simulink model "wlan_mac_hw"  (Simulink 7.8)
settings: Solver=ode45  StartTime=0.0  StopTime=200  RelTol=1e-3
PostLoadFcn:
  | wlan_mac_hw_init
InitFcn:
  | wlan_mac_hw_init
StartFcn:
  | wlan_mac_hw_init
values from neighbouring files (symbols this model uses):
  NB_CNTR_NAV = ceil(log2(MAX_NAV * 160))    [wlan_mac_hw_init.m]
  ticks_per_usec = 10    [wlan_mac_hw_init.m]
undefined symbols (not defined in the file or in its folder): gcbh, xlBlockLoadCallback, xlGetNormalizedPeriod
libraries: xbsIndex_r4 x788, xbsEDKLib_r4 x1
(part 1 of 6)
settings Model: Creator=murphpo  LastModifiedBy=murphpo
settings DebuggingCC: SolverPrmCheckMsg=none  InheritedTsInSrcMsg=none  UnconnectedInputMsg=none  UnconnectedOutputMsg=none  UnconnectedLineMsg=none

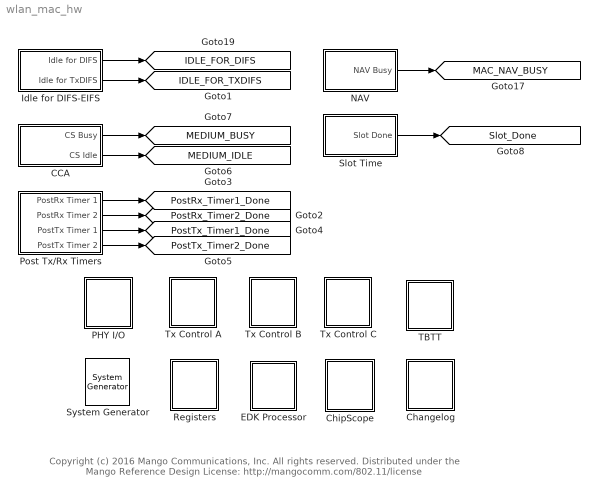
== system wlan_mac_hw ==
  note: Copyright (c) 2016 Mango Communications, Inc. All rights reserved.
      |
      | Distributed under the Mango Reference Design License:
      | http://mangocomm.com/802.11/license
  " System Generator" : xbsIndex_r4/ System Generator  Tag=genX  xilinxfamily=virtex6  part=xc6vlx240t  speed=-2  package=ff1156  synthesis_tool=XST  clock_wrapper=Clock Enables  directory=./pcore_v212  proj_type=Project Navigator  Synth_file=XST Defaults  Impl_file=ISE Defaults  testbench=off  simulink_period=1  sysclk_period=10  dcm_input_clock_period=10  incr_netlist=off  trim_vbits=Everywhere in SubSystem  dbl_ovrd=According to Block Masks  core_generation=According to Block Masks  run_coregen=off  deprecated_control=off  eval_field=0  block_type=sysgen
  CCA : Subsystem
  Changelog : Subsystem
  ChipScope : Subsystem
  EDK Processor : Subsystem  LoadFcn=xlBlockLoadCallback(gcbh);  mask(Xilinx EDK Processor Block){mode=EDK pcore generation, xmp=, MemVisToProc=<qt bgcolor="#FFFFFF"><div><img src="S:/Xilinx/14.4/ISE_DS/ISE/sysgen/data/images/registerplus.gif"> &lt;&lt;TX_CTRL_B_PARAMS&gt;&gt;<br></div><div><img src="S:/Xilinx/14.4/ISE_DS/ISE/sysgen/data/images/registerplus.gif"> &lt;&lt;TX_CTRL_A_GAINS&gt;&gt;<br></div><div><img src="S:/Xilinx/14.4/ISE_DS/ISE/sysgen/data/images/registerplus.gif"> &lt;&lt;TX_CTRL_C_PARAMS&gt;&gt;<br></div><div><img src="S:/Xilinx/14.4/ISE_DS/ISE/sysgen/data/images/registerplus.gif"> &lt;&lt;TX_CTRL_A_PARAMS&gt;&gt;<br></div><div><img src="S:/Xilinx/14.4/ISE_DS/ISE/sysgen/data/images/registerplus.gif"> &lt;&lt;TX_CTRL_C_GAINS&gt;&gt;<br></div><div><img src="S:/Xilinx/14.4/ISE_DS/ISE/sysgen/data/images/registerplus.gif"> &lt;&lt;POST_RX_TIMERS&gt;&gt;<br></div><div><img src="S:/Xilinx/14.4/ISE_DS/ISE/sysgen/data/images/registerplus.gif"> &lt;&lt;TX_CTRL_B_GAINS&gt;&gt;<br></div><div><img src="S:/Xilinx/14.4/ISE_DS/ISE/sysgen/data/images/registerplus.gif"> &lt;&lt;POST_TX_TIMERS&gt;&gt;<br></div><div><img src="S:/Xilinx/14.4/ISE_DS/ISE/sysgen/data/images/registerplus.gif"> &lt;&lt;CALIB_TIMES&gt;&gt;<br></div><div><img src="S:/Xilinx/14.4/ISE_DS/ISE/sysgen/data/images/registerplus.gif"> &lt;&lt;IFS_INTERVALS2&gt;&gt;<br></div><div><img src="S:/Xilinx/14.4/ISE_DS/ISE/sysgen/data/images/registerplus.gif"> &lt;&lt;IFS_INTERVALS1&gt;&gt;<br></div><div><img src="S:/Xilinx/14.4/ISE_DS/ISE/sysgen/data/images/registerplus.gif"> &lt;&lt;TX_START&gt;&gt;<br></div><div><img src="S:/Xilinx/14.4/ISE_DS/ISE/sysgen/data/images/registerplus.gif"> &lt;&lt;TU_TARGET&gt;&gt;<br></div><div><img src="S:/Xilinx/14.4/ISE_DS/ISE/sysgen/data/images/registerplus.gif"> &lt;&lt;Control&gt;&gt;<br></div><div><img src="S:/Xilinx/14.4/ISE_DS/ISE/sysgen/data/images/registerplus.gif"> &lt;&lt;NAV_MATCH_ADDR_1&gt;&gt;<br></div><div><img src="S:/Xilinx/14.4/ISE_DS/ISE/sysgen/data/images/registerplus.gif"> &lt;&lt;NAV_MATCH_ADDR_2&gt;&gt;<br></div><div><img src="S:/Xilinx/14.4/ISE_DS/ISE/sysgen/data/images/registerplus.gif"> &lt;&lt;BACKOFF_CTRL&gt;&gt;<br></div><div><img src="S:/Xilinx/14.4/ISE_DS/ISE/sysgen/data/images/registerplus.gif"> &lt;&lt;NAV_VALUE&gt;&gt;<br></div><div><img src="S:/Xilinx/14.4/ISE_DS/ISE/sysgen/data/images/registerplus.gif"> &lt;&lt;BACKOFF_COUNTERS&gt;&gt;<br></div><div><img src="S:/Xilinx/14.4/ISE_DS/ISE/sysgen/data/images/registerplus.gif"> &lt;&lt;PHY_RX_PARAMS&gt;&gt;<br></div><div><img src="S:/Xilinx/14.4/ISE_DS/ISE/sysgen/data/images/registerplus.gif"> &lt;&lt;LATEST_RX_BYTE&gt;&gt;<br></div><div><img src="S:/Xilinx/14.4/ISE_DS/ISE/sysgen/data/images/registerplus.gif"> &lt;&lt;TX_START_TIMESTAMP_MSB&gt;&gt;<br></div><div><img src="S:/Xilinx/14.4/ISE_DS/ISE/sysgen/data/images/registerplus.gif"> &lt;&lt;TX_START_TIMESTAMP_LSB&gt;&gt;<br></div><div><img src="S:/Xilinx/14.4/ISE_DS/ISE/sysgen/data/images/registerplus.gif"> &lt;&lt;RX_START_TIMESTAMP_MSB&gt;&gt;<br></div><div><img src="S:/Xilinx/14.4/ISE_DS/ISE/sysgen/data/images/registerplus.gif"> &lt;&lt;RX_START_TIMESTAMP_LSB&gt;&gt;<br></div><div><img src="S:/Xilinx/14.4/ISE_DS/ISE/sysgen/data/images/registerplus.gif"> &lt;&lt;TXRX_START_TIMESTAMPS_FRAC&gt;&gt;<br></div><div><img src="S:/Xilinx/14.4/ISE_DS/ISE/sysgen/data/images/registerplus.gif"> &lt;&lt;Status&gt;&gt;<br></div></qt>, AvailableMemories=<empty>, portInterfaceTable={'exposed'=>[],'portdir'=>[],'portname'=>[],'shortname'=>[]}, bus_type_sgadvanced=, bus_type=AXI, baseaddr=0x80000000, baseaddr_lock_sgadvanced=, baseaddr_lock=off, dual_clock_sgadvanced=, dual_clock=on, reg_readback_sgadvanced=, reg_readback=on, ucf_file=, inheritDeviceType_sgadvanced=, inheritDeviceType=off, elf_file=, codebug_sgadvanced=, codebug=on, clock_name=plb, internalPortList={}, resetPolarity=0, memxtable=|, procinfo={}, memmapdirty=off, blockname=, xpsintstyle=default, has_advanced_control=0, sggui_pos=-1,-1,-1,-1, block_type=edkprocessor, block_version=2.7, sg_icon_stat=42,45,-1,-1,white,blue,0,07734,right,,[ ],[ ], sg_mask_display=|, sg_list_contents={'table'=>{'AvailableMemories'=>'popup(<empty>)'}}, sg_blockgui_xml=}
      mask memxtable=|
      | {'mladdr'=>[0.00000000000000000,1.00000000000000000,2.00000000000000000,3.00000000000000000,4.00000000000000000,5.00000000000000000,6.00000000000000000,7.00000000000000000,8.00000000000000000,9.00000000000000000,10.00000000000000000,11.00000000000000000,12.00000000000000000,13.00000000000000000,14.00000000000000000,15.00000000000000000,16.00000000000000000,0.00000000000000000,1.00000000000000000,2.00000000000000000,3.00000000000000000,4.00000000000000000,5.00000000000000000,6.00000000000000000,7.00000000000000000,8.00000000000000000,9.00000000000000000],'mlist'=>['wlan_mac_hw/Registers/Tx Controller
      | Regs/From Register9','wlan_mac_hw/Registers/Tx Controller
      | Regs/From Register7','wlan_mac_hw/Registers/Tx Controller
      | Regs/From Register4','wlan_mac_hw/Registers/Tx Controller
      | Regs/From Register3','wlan_mac_hw/Registers/Tx Controller
      | Regs/From Register2','wlan_mac_hw/Registers/Tx Controller
      | Regs/From Register14','wlan_mac_hw/Registers/Tx Controller
      | Regs/From Register12','wlan_mac_hw/Registers/Tx Controller
      | Regs/From Register1','wlan_mac_hw/Registers/From Register8','wlan_mac_hw/Registers/From Register6','wlan_mac_hw/Registers/From Register5','wlan_mac_hw/Registers/From Register4','wlan_mac_hw/Registers/From Register3','wlan_mac_hw/Registers/From Register2','wlan_mac_hw/Registers/From Register16','wlan_mac_hw/Registers/From Register15','wlan_mac_hw/Registers/From Register1','wlan_mac_hw/Registers/To Register7','wlan_mac_hw/Registers/To Register4','wlan_mac_hw/Registers/To Register2','wlan_mac_hw/Registers/To Register1','wlan_mac_hw/Registers/Timestamp
      | Regs & IO/To Register9','wlan_mac_hw/Registers/Timestamp
      | Regs & IO/To Register8','wlan_mac_hw/Registers/Timestamp
      | Regs & IO/To Register6','wlan_mac_hw/Registers/Timestamp
      | Regs & IO/To Register5','wlan_mac_hw/Registers/Timestamp
      | Regs & IO/To Register1','wlan_mac_hw/Registers/Status Register/To Register'],'mlname'=>['\\'TX_CTRL_B_PARAMS\\'','\\'TX_CTRL_A_GAINS\\'','\\'TX_CTRL_C_PARAMS\\'','\\'TX_CTRL_A_PARAMS\\'','\\'TX_CTRL_C_GAINS\\'','\\'POST_RX_TIMERS\\'','\\'TX_CTRL_B_GAINS\\'','\\'POST_TX_TIMERS\\'','\\'CALIB_TIMES\\'','\\'IFS_INTERVALS2\\'','\\'IFS_INTERVALS1\\'','\\'TX_START\\'','\\'TU_TARGET\\'','\\'Control\\'','\\'NAV_MATCH_ADDR_1\\'','\\'NAV_MATCH_ADDR_2\\'','\\'BACKOFF_CTRL\\'','\\'NAV_VALUE\\'','\\'BACKOFF_COUNTERS\\'','\\'PHY_RX_PARAMS\\'','\\'LATEST_RX_BYTE\\'','\\'TX_START_TIMESTAMP_MSB\\'','\\'TX_START_TIMESTAMP_LSB\\'','\\'RX_START_TIMESTAMP_MSB\\'','\\'RX_START_TIMESTAMP_LSB\\'','\\'TXRX_START_TIMESTAMPS_FRAC\\'','\\'Status\\''],'mlstate'=>[0.00000000000000000,0.00000000000000000,0.00000000000000000,0.00000000000000000,0.00000000000000000,0.00000000000000000,0.00000000000000000,0.00000000000000000,0.00000000000000000,0.00000000000000000,0.00000000000000000,0.00000000000000000,0.00000000000000000,0.00000000000000000,0.00000000000000000,0.00000000000000000,0.00000000000000000,0.00000000000000000,0.00000000000000000,0.00000000000000000,0.00000000000000000,0.00000000000000000,0.00000000000000000,0.00000000000000000,0.00000000000000000,0.00000000000000000,0.00000000000000000]}
      mask sg_mask_display=|
      | fprintf('','COMMENT: begin icon graphics');
      | patch([0 42 42 0 0 ],[0 0 45 45 0 ],[0.77 0.82 0.91 ]);
      | plot([0 42 42 0 0 ],[0 0 45 45 0 ]);
      | patch([7.65 16.32 22.32 28.32 34.32 22.32 13.65 7.65 ],[28.66 28.66 34.66 28.66 34.66 34.66 34.66 28.66 ],[1 1 1 ]);
      | patch([13.65 22.32 16.32 7.65 13.65 ],[22.66 22.66 28.66 28.66 22.66 ],[0.931 0.946 0.973 ]);
      | patch([7.65 16.32 22.32 13.65 7.65 ],[16.66 16.66 22.66 22.66 16.66 ],[1 1 1 ]);
      | patch([13.65 34.32 28.32 22.32 16.32 7.65 13.65 ],[10.66 10.66 16.66 10.66 16.66 16.66 10.66 ],[0.931 0.946 0.973 ]);
      | fprintf('','COMMENT: end icon graphics');
      | fprintf('','COMMENT: begin icon text');
      | fprintf('','COMMENT: end icon text');
      mask prompts: mode "Configure Processor for"; xmp "XPS Project"; MemVisToProc ""; AvailableMemories "Available Memories"; portInterfaceTable ""; bus_type_sgadvanced ""; bus_type "Bus Type"; baseaddr "Base Address"; baseaddr_lock_sgadvanced ""; baseaddr_lock "Lock"; dual_clock_sgadvanced ""; dual_clock "Dual Clocks"; reg_readback_sgadvanced ""; reg_readback "Register Read-Back"; ucf_file "Constraint File"; inheritDeviceType_sgadvanced ""; inheritDeviceType "Inherit Device Type"; elf_file "Initial Program"; codebug_sgadvanced ""; codebug "Enable Co-Debug with Xilinx SDK (Beta)"; clock_name ""; internalPortList ""; resetPolarity ""; memxtable ""; procinfo ""; memmapdirty ""; blockname ""; xpsintstyle ""; has_advanced_control ""; sggui_pos ""; block_type ""; block_version ""; sg_icon_stat ""; sg_mask_display ""; sg_list_contents ""; sg_blockgui_xml ""
      mask help: Xilinx EDK Processor
      mask init:
      | try
      |   tmp_gcb = gcb;
      |   tmp_gcbh = gcbh;
      |   if (strcmp('SysGenIndex',get_param(bdroot(tmp_gcbh),'tag')) && ~isempty(regexp(bdroot(tmp_gcb), '^xbs', 'once')))
      |     return;
      |   end;
      |   xlMungeMaskParams;
      | 
      |   block_type='edkprocessor';
      | 
      |   serialized_declarations = '{''block_type''=>''String''}';
      |   xledkprocessor_init();
      |   ptable_ = xlblockprep(get_param(tmp_gcb, 'MaskWSVariables'));
      |   try
      |     xlBlockMoveCallback(tmp_gcbh);
      |   catch 
      |      clear global xl_updateicon_recursion_guard;
      |   end;
      | catch
      |   global dbgsysgen;
      |   if(~isempty(dbgsysgen) && dbgsysgen)
      |     e = regexprep(lasterr, '\n', '\nError: ');
      |     disp(['Error: While running MaskInit code on block ' tmp_gcb ': ' e]);
      |     error(e);
      |   end
      | end
      settings: CopyFcn=xlProcBlockCopyCallback(gcbh);xlBlockMoveCallback(gcbh);  DeleteFcn=xlDestroyGui(gcbh);  ModelCloseFcn=xlDestroyGui(gcbh);  PreSaveFcn=xlBlockPreSaveCallback(gcbh);  PostSaveFcn=xlBlockPostSaveCallback(gcbh);  DestroyFcn=xlDestroyGui(gcbh);  OpenFcn=bh=gcbh;xlProcBlockCallbacks('populatesharedmemorylistbox',bh);xlOpenGui(bh, 'edkprocessor_gui.xml', @xlProcBlockEnablement, @xlProcBlockAction);  CloseFcn=xlDestroyGui(gcbh);  MoveFcn=xlBlockMoveCallback(gcbh);
      mask Help: eval('');xlDoc('-book','sysgen','-topic','EDK_Processor');
      mask StyleString: popup(EDK pcore generation|HDL netlisting),edit,edit,edit,edit,edit,popup(AXI|PLB),edit,edit,checkbox,edit,checkbox,edit,checkbox,edit,edit,checkbox,edit,edit,checkbox,edit,edit,edit,edit,edit,edit,edit,edit,edit,edit,edit,edit,edit,edit,edit,edit
      mask Display:
      | fprintf('','COMMENT: begin icon graphics');
      | patch([0 42 42 0 0 ],[0 0 45 45 0 ],[0.77 0.82 0.91 ]);
      | plot([0 42 42 0 0 ],[0 0 45 45 0 ]);
      | patch([7.65 16.32 22.32 28.32 34.32 22.32 13.65 7.65 ],[28.66 28.66 34.66 28.66 34.66 34.66 34.66 28.66 ],[1 1 1 ]);
      | patch([13.65 22.32 16.32 7.65 13.65 ],[22.66 22.66 28.66 28.66 22.66 ],[0.931 0.946 0.973 ]);
      | patch([7.65 16.32 22.32 13.65 7.65 ],[16.66 16.66 22.66 22.66 16.66 ],[1 1 1 ]);
      | patch([13.65 34.32 28.32 22.32 16.32 7.65 13.65 ],[10.66 10.66 16.66 10.66 16.66 16.66 10.66 ],[0.931 0.946 0.973 ]);
      | fprintf('','COMMENT: end icon graphics');
      | fprintf('','COMMENT: begin icon text');
      | disp('');
      | 
      | fprintf('','COMMENT: end icon text');
  Idle for DIFS-EIFS : Subsystem
  NAV : Subsystem
  PHY I/O : Subsystem
  Post Tx/Rx Timers : Subsystem
  Registers : Subsystem
  Slot Time : Subsystem
  TBTT : Subsystem
  Tx Control A : Subsystem
  Tx Control B : Subsystem
  Tx Control C : Subsystem
  tag scope: IDLE_FOR_DIFS=global, IDLE_FOR_TXDIFS=global, MAC_NAV_BUSY=global, MEDIUM_BUSY=global, MEDIUM_IDLE=global, PostRx_Timer1_Done=global, PostRx_Timer2_Done=global, PostTx_Timer1_Done=global, PostTx_Timer2_Done=global, Slot_Done=global
  wires:
  Idle for DIFS-EIFS/1(Idle for DIFS) -> [IDLE_FOR_DIFS]
  NAV/1(NAV Busy) -> [MAC_NAV_BUSY]
  CCA/1(CS Busy) -> [MEDIUM_BUSY]
  Idle for DIFS-EIFS/2(Idle for TxDIFS) -> [IDLE_FOR_TXDIFS]
  CCA/2(CS Idle) -> [MEDIUM_IDLE]
  Post Tx/Rx Timers/1(" PostRx Timer 1") -> [PostRx_Timer1_Done]
  Post Tx/Rx Timers/2(" PostRx Timer 2") -> [PostRx_Timer2_Done]
  Post Tx/Rx Timers/3(" PostTx Timer 1") -> [PostTx_Timer1_Done]
  Post Tx/Rx Timers/4(" PostTx Timer 2") -> [PostTx_Timer2_Done]
  Slot Time/1(Slot Done) -> [Slot_Done]

== system wlan_mac_hw/CCA ==
  note: Medium is busy if:
      |
      | PHY Tx is running
      | OR
      | PHY Rx indicates CCA Busy
      | OR
      | MAC NAV indicates Busy
  Inverter{1..4} (4 alike) : xbsIndex_r4/Inverter  en=off  latency=0  dbl_ovrd=off  block_type=inv
      settings: xl_area=[0 0 0 0 0 0 0]  block_version=VER_STRING_GOES_HERE
  Logical1 : xbsIndex_r4/Logical  logical_function=AND  inputs=2  en=off  latency=0  precision=Full  arith_type=Unsigned  n_bits=16  bin_pt=0  align_bp=on  dbl_ovrd=off  block_type=logical
  Logical2 : xbsIndex_r4/Logical  logical_function=AND  inputs=2  en=off  latency=0  precision=Full  arith_type=Unsigned  n_bits=16  bin_pt=0  align_bp=on  dbl_ovrd=off  block_type=logical
  Logical3 : xbsIndex_r4/Logical  logical_function=OR  inputs=4  en=off  latency=0  precision=Full  arith_type=Unsigned  n_bits=16  bin_pt=0  align_bp=on  dbl_ovrd=off  block_type=logical
  Logical4 : xbsIndex_r4/Logical  logical_function=AND  inputs=2  en=off  latency=0  precision=Full  arith_type=Unsigned  n_bits=16  bin_pt=0  align_bp=on  dbl_ovrd=off  block_type=logical
  CS Busy : Outport
  CS Idle : Outport  Port=2
  wires:
  Logical3/1 -> CS Busy/1, Inverter1/1
  Inverter1/1 -> CS Idle/1
  [MAC_NAV_BUSY] -> Logical1/1
  [reg_CCA_Ignore_NAV] -> Inverter4/1
  [PHY_CCA_IND_BUSY] -> Logical2/1
  [reg_CCA_Ignore_PHY_CS] -> Inverter3/1
  [Status_Tx_PHY_Active] -> Logical4/1
  [reg_CCA_Ignore_TxBusy] -> Inverter2/1
  Inverter2/1 -> Logical4/2
  Inverter3/1 -> Logical2/2
  Inverter4/1 -> Logical1/2
  Logical4/1 -> Logical3/1
  Logical2/1 -> Logical3/2
  Logical1/1 -> Logical3/3
  [reg_CCA_Force_Busy] -> Logical3/4

== system wlan_mac_hw/Changelog ==
  note: 1.00.e:
      | Reworked backoff state to allow numSlots=0 at backoff start,
      | finishing at next idle_for_difs
      |
      | 1.00.f:
      | Same as 1.00.e, with ILA removed (to allow ILA in PHY)
      |
      | 1.00.g:
      | -Changed auto_tx logic to check auto_tx_en after TxSIFS counter
      |   finishes, for extra MAC processing time
      | -Renamed from/goto/regs for MPDU Tx logic
      | -Re-enabled ILA
      |
      | 1.00.h:
      | -Removed ILA
      | -Added FCS_GOOD to status reg
      |
      | 1.00.i:
      | -Added logic to block Rx pkt det (replacement for Rx PHY blocking pkt done)
      | -Added rate_length register with SIGNAL.rate, length and PHY_SEL captured
      |   at RX_START
      |
      | 1.00.j:
      | -Blocked on FCS_Good now gated by data_done, not rx_end
      |
      | 1.00.k:
      | -Added gw outs for 64-bit timestamp
      | -Added SR latch for auto-tx-en, so each assertion results in (at most) 1 auto Tx event
      |
      | 1.00.l:
      | -Added reg reset in front of last_byte_rx reg so last_byte_rx_index = 0 at every rx start
      |
      | 1.00.m:
      | -Fixed backoff start bug when IDLE_FOR_DIFS = 1
      |
      | 1.00.n:
      | -Fixed byte order for capturing NAV duration
      | -Added debug outputs
      |
      | 1.00.o:
      | -Added option to not block Rx on Tx_Active (trying to debug odd Rx states...)
      |
      | 1.00.p:
      | -Added delay from RX_START_IND to status register, so Tx MPDU FSM has time
      |   to react to new Rx before MAC code notices
      | -Fixed checking of backoff_done by MPDU FSM - now FSM-initiated backoff will properly
      |   cause deferral of FSM-initiated Tx
      |
      | 1.00.q:
      | -Moved block_rx condition to rx_end & fcs_good from data_done & fcs_good (to avoid blocking
      |   rx phy while it's still in the post-last-byte extension, which lead to incorrect rx_end.error events)
      |
      | 1.00.r:
      | -Added time_at_rx_start registers (64-bit total)
      |
      | 1.00.s:
      | -Added backoff decrement logging via bram_block interface
      |
      | 1.00.t:
      | -Added option to block PHY Rx on all RxStart->RxEnd events, to preserve bad-FCS pkts for logging
      |
      | 1.00.u:
      | -Added BO pending logic, so node gets credit for starting 0-slot backoff during DIFS interval
      | -Cleaned up IFS registers
      | -Changed NAV_Adj value to Fix8_0 (was UFix10_0) to allow negative adjustment times
      | -Removed unused reset input
      |
      | 1.00.v:
      | -Reverted unnecessary backoff control change (old logic correctly handled zero backoff case)
      |
      | 1.00.w:
      | -Removed unused "Logging" subsystem (still trying to figure out best way to log backoff trace)
      | -Added NAV value register so software can check current NAV counter
  note: 1.00.x:
      | Added TxGain params to MPDU Tx and Auto Tx paths, captured and output to PHY for per-pkt Tx pwr control
      | Added TX_START_TIMESTAMP registers
      |
      | 1.00.y:
      | Added posedge's to timestamp capture register enables
      |   (1.00.x TX_START was "enbaled" for whole pkt, instead of once at TX_START)
      |
      | 1.00.z:
      | Added software resets for NAV and backoff counters (not required by standard, but useful for research)
      |
      | 1.01.a:
      | Added TX_START time output for PHY Tx timestamp insertion (better than inserting raw timestamp)
      |
      | 1.01.b:
      | Added RX_ERROR==0 as condition for blocking on FCS_Good
      |
      | 1.01.c-e:
      | Added register to add/subtract value from TX_START timestampe output. This offset adjusts the timestamp
      |  value inserted into transmitted beacons, compensating for Tx latencies betwee Tx start and actual Tx.
      |
      | 1.01.f:
      | Increased backoff slot counter to 16 bits, matching num_slots values in Tx config registers. NOTE: This
      |   change modified the bit assignments in the STATUS register. The MAC software macros must be updated
      |   to match.
      |
      | 2.00.a:
      | Generalized Tx control state machines (A and B replace MPDU_Tx and Auto_Tx); hardware now supports
      |   complicated pkt exchanges like RTS/CTS/DATA/ACK and DATA/DATA/.../ACK
      | Dropped _dcf from core name
      | Added addressed-to-me exclusion for NAV update
      |
      | 2.00.b:
      | Added reset bits for each Tx controller FSM in control register
      | Removed the 64-bit microsecond counter (to be part of new wlan_mac_time_hw core)
      | Added new gateways for timestamp input, to be captured on Tx/Rx start events, as before
      |
      | 2.00.c:
      | Added Tx_Inhibit input, logic and register
      |
      | 2.00.d:
      | Added per-FSM reset to OR for TX_PENDING bit in each Tx subsystem; without this PENDING would not
      |   de-assert on the FSM reset, leading to a never-Tx-again state in software
      |
      | 2.00.e:
      | Added MAC_TIME_USEC_FRAC input and register with FRAC value captured at Tx/Rx start
      |
      | 2.00.f:
      | Fixed differing latencies between integer and fractional parts of Tx/Rx start timestamps
      |
      | 2.01.a:
      | -Added Tx C controller, designed for transmtting beacons, possibly while Tx A is deferring
      | -Updated PHY Tx interface for new Tx core, with 11n support
      | -Promoted slot timer to top-level block
      | -Demoted backoff to inside Tx A controller, added separate backoff for Tx C controller. Both backoff
      |   counters use common slot timer
      | -Added "C not pending" condition to A backoff decrement (required to transmit beacons during Tx A deferral)
      | -Added "software CCA busy" bit, so code can fake busy medium any time
      | -Removed TX_START_TIMESTAMP outputs; Tx PHY doesn't use these anymore
      |
      | 2.01.b:
      | -Added TBTT subsystem with simple Target_TU > Current_TU circuit

== system wlan_mac_hw/ChipScope ==
  4-bit Count : xbsIndex_r4/Counter  cnt_type=Free Running  cnt_to=Inf  operation=Up  start_count=0  cnt_by_val=1  arith_type=Unsigned  n_bits=4  bin_pt=0  load_pin=off  rst=off  en=off  explicit_period=on  period=1  dbl_ovrd=off  use_behavioral_HDL=off  implementation=Fabric  block_type=counter
  ChipScope : xbsIndex_r4/ChipScope  num_trig_ports=15  current_port=9  show_trig_port=0  match_units=1  match_type=Basic with edges  data_is_trigger=on  num_data_ports=1  data_depth=4096  SRL16s=on  add_bufg=on  match_type_t0=2  match_type_t1=2  match_type_t2=2  match_type_t3=2  match_type_t4=2  match_type_t5=2  match_type_t6=2  match_type_t7=2  match_type_t8=2  match_type_t9=2  match_type_t10=1  match_type_t11=1  match_type_t12=1  match_type_t13=1  match_type_t14=1  match_type_t15=1  match_units_t0=1  match_units_t1=1  match_units_t2=1  match_units_t3=1  match_units_t4=1  match_units_t5=1  match_units_t6=1  match_units_t7=1  match_units_t8=1  match_units_t9=1  match_units_t10=1  match_units_t11=1  match_units_t12=1  match_units_t13=1  match_units_t14=1  match_units_t15=1  dbl_ovrd=0  user_scan_chain=USER1  block_type=chipscope
      settings: infoedit="Enables run-time debugging and verification of signals by inserting ChipScope Pro ICON and ILA cores.<br><br>  Restrictions: <br>Only one ChipScope core can be instantiated in a System Generator design. A design or subsystem containing a ChipScope block must have at least one output port."
  Disregard Subsystem : xbsIndex_r4/Disregard Subsystem  Tag=discardX  block_type=disregard
  Register : xbsIndex_r4/Register  init=0  rst=off  en=on  dbl_ovrd=off  block_type=register
  Register1 : xbsIndex_r4/Register  init=0  rst=off  en=on  dbl_ovrd=off  block_type=register
  Register{2..13} (12 alike) : xbsIndex_r4/Register  init=0  rst=off  en=off  dbl_ovrd=off  block_type=register
  wires:
  [Tx_A_PHY_Start] -> Register2/1
  [Tx_B_PHY_Start] -> Register3/1
  [reg_status] -> Register4/1
  [PostRx_Timer1_Done] -> Register5/1
  [Tx_A_Backoff_Start] -> Register6/1
  [PHY_RX_FCS_GOOD_IND] -> Register7/1
  [PHY_RX_START_IND] -> Register8/1
  [PHY_RX_END_IND] -> Register9/1
  [PHY_RX_END_RXERROR] -> Register10/1
  [PHY_CCA_IND_BUSY] -> Register11/1
  [MAC_NAV_BUSY] -> Register12/1
  [Status_Tx_PHY_Active] -> Register13/1
  Register/1 -> ChipScope/14  "Rx Byte Ind"
  [PHY_RX_BYTENUM] -> Register/1
  Register1/1 -> ChipScope/15  "Rx Byte"
  [PHY_RX_BYTE] -> Register1/1
  [PHY_RX_BYTE_VALID] -> Register/2, Register1/2
  Register2/1 -> ChipScope/2  "New Tx PHY Start"
  Register3/1 -> ChipScope/3  "Auto Tx PHY Start"
  Register4/1 -> ChipScope/4  "Status Reg"
  Register5/1 -> ChipScope/5  "Post Rx Timer 1 Done"
  Register6/1 -> ChipScope/6  "Tx Backoff Start"
  Register7/1 -> ChipScope/7  "FCS Good"
  Register8/1 -> ChipScope/8  "PHY Rx Start"
  Register9/1 -> ChipScope/9  "PHY Rx End"
  Register10/1 -> ChipScope/10  "PHY Rx End Error"
  Register11/1 -> ChipScope/11  "PHY CCA Busy"
  Register12/1 -> ChipScope/12  "NAV Busy"
  Register13/1 -> ChipScope/13  "Tx Active"
  4-bit Count/1 -> ChipScope/1  "Trig Counter"
